simulink model "Copy_of_Channalizer_smoke_tmp"  (R2024a)
settings: Solver=VariableStepAuto  StartTime=0.0  StopTime=500  RelTol=1e-3
values from neighbouring files (symbols this model uses):
  X = simout    [outputPlots.m]
undefined symbols (not defined in the file or in its folder): Configured, DVB, es1, F, Initialized_retain_I, Pre, S, S2, vsva2488, xcvr1602
libraries: hdlBasic x21, hdlDSPIP x1, vmcUtilities x1
settings Model: Creator=nanumolu  LastModifiedBy=nanumolu

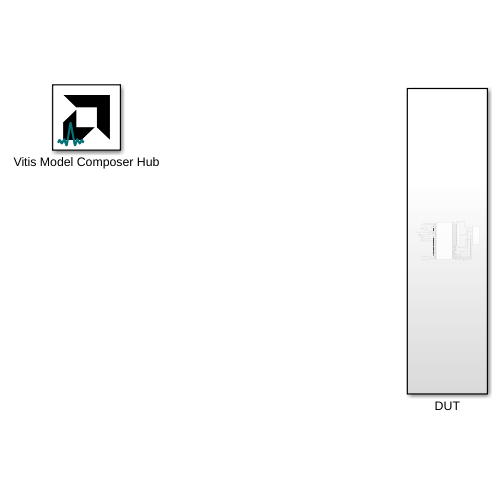
[thumbnail: Simulink's stored preview of the top-level diagram]
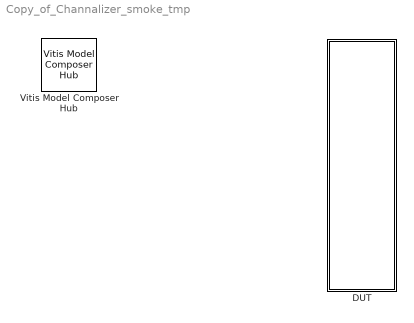
== system Copy_of_Channalizer_smoke_tmp ==
  DUT : Subsystem
  Vitis Model Composer Hub : vmcUtilities/Vitis Model Composer Hub  Tag=genX  CodeGeneration=off  SubsystemName=Channalizer_smoke_tmp  BlockHierPath=Channalizer_smoke_tmp  CompilationType=HDLCompilation  SubsystemType=HDLNode  ExportTypeV2=HDL Netlist  StartColumn=1  NumberOfColumns=1  TargetDirectory=./netlist_ldpc_vhd  exportDesign=on  analyzeDesign=off  validateDesignOnHw=off  ExportType=AI Engines  IpVendor=xilinx.com  IpLibrary=hls  IpVersion=1.0  IpHWLanguage=Verilog  AieCompilerOptions={}  AieSimulatorOptions={}  CreateTestbench=on  TestbenchStackSize=10  RunRtlSim=off  RunCSim=off  RunAieSim=off  AieSimTimeout=50000  RunAieSimProfiling=off  LaunchVitisAnalyzer=off  PlotOutput=off  RunX86Sim=off  X86SimTimeout=10  GenHwImage=off  GenLibadfXo=off  GenHwValidationCode=off  PlatformType=Not Specified  HwSystemType=Baremetal  HwValidationTarget=hw  ProjDevice=xcvr1602-vsva2488-2MP-e-S-es1  ProjDevicePart=xcvr1602-vsva2488-2MP-e-S-es1  AIEType=AIE  SamplePeriod=-1  ClockFrequency=200  DataPathParallelism=1  xilinxfamily=versalairfes1  part=xcvr1602  speed=-2MP-e-S-es1  package=vsva2488  directory=./netlist_ldpc_vhd  testbench=on  incr_netlist=off  synthesis_tool=Vivado  clock_wrapper=Clock Enables  dbl_ovrd=According to Block Masks  dcm_input_clock_period=10  sysclk_period=10  simulink_period=1  eval_field=0  IPInfoJsonString="{\"DUTSubsystemName\":\"Channalizer_smoke_tmp\",\"HDLSubsystem\":{\"SubsystemName\":\"Channalizer_smoke_tmp\",\"IPName\":\"Copy_of_hamilton_vrf_fft\",\"IPLibrary\":\"VMC\",\"IPVendor\":\"User Company\",\"IPVersion\":\"1.0\",\"TargetDirectory\":\"./netlist_ldpc_vhd\",\"SubsystemDir\":\"./netlist_ldpc_vhd/ip/Channalizer_smoke_tmp\",\"FreqHz\":\"100000000\"},\"SubsystemTag\":\"HDLNode\"}"  LogFileName=/proj/xhdhdstaff2/nanumolu/test/modelcomposer/hdl/regression/blocks/ip/RF_channelizer/smoke/Channalizer_smoke/netlist_ldpc_vhd/model_composer.log  NThreads=4  IPConfigFile=/tmp/vmctmp-3516168675900120850/Channalizer_smoke_tmp_ipconfig.json

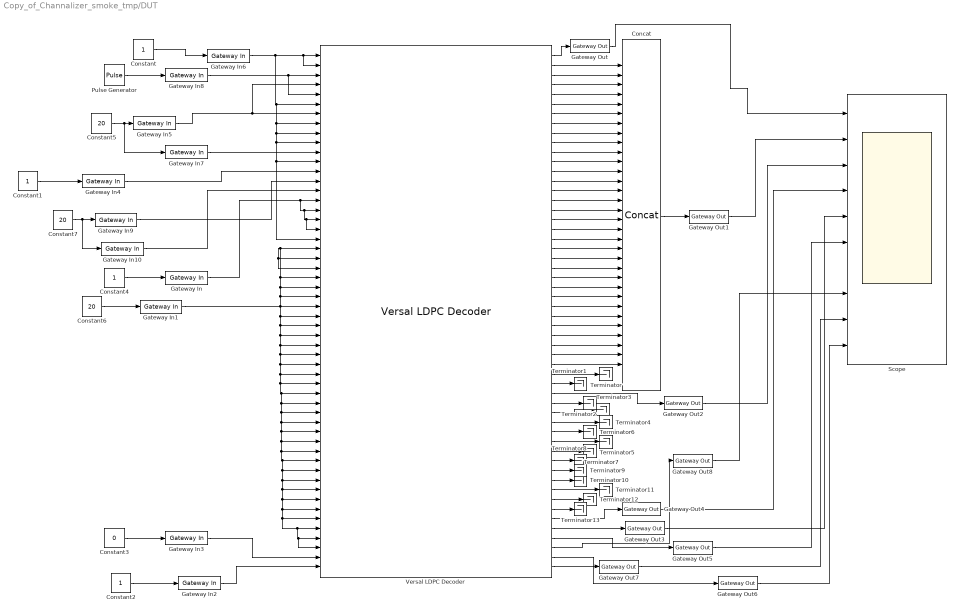
== system Copy_of_Channalizer_smoke_tmp/DUT ==
  Concat : hdlBasic/Concat  num_inputs=32  XmcBlockStatus=1  maskContainerNames=group1  block_type=concat  block_config=sysgen:Concat_config
  Constant : Constant  SampleTime=1/1e4
  Constant1 : Constant  SampleTime=1/1e4
  Constant2 : Constant  SampleTime=1
  Constant3 : Constant  Value=0  SampleTime=1
  Constant4 : Constant  SampleTime=1/1e4
  Constant5 : Constant  Value=20  SampleTime=1/1e4
  Constant6 : Constant  Value=20  SampleTime=1/1e4
  Constant7 : Constant  Value=20  SampleTime=1/1e4
  Gateway In : hdlBasic/Gateway In  gui_display_data_type=Fixed-point  arith_type=Unsigned  n_bits=1  bin_pt=0  preci_type=Single  exp_width=8  frac_width=24  rows=1  columns=1  quantization="Round  (unbiased: +/- Inf)"  overflow=Saturate  period=1  UseAsADC=off  ADCChannel='1'  interface=None  automatic_assignment=on  address_offset=hex2dec('00')  intf_name=''  intf_description=''  default_value=0  timing_constraint=None  locs_specified=off  LOCs={}  io_standard={}  inherit_from_input=off  hdl_port=on  XmcBlockStatus=1  maskContainerNames=group4  block_type=gatewayin  block_config=sysgen:gateway_in_config  block_width_w=590  block_height_w=620  block_width=640  block_height=850
  Gateway In1 : hdlBasic/Gateway In  gui_display_data_type=Fixed-point  arith_type=Signed (2's comp)  n_bits=8  bin_pt=2  preci_type=Single  exp_width=8  frac_width=24  rows=1  columns=1  quantization="Round  (unbiased: +/- Inf)"  overflow=Saturate  period=1  UseAsADC=off  ADCChannel='1'  interface=None  automatic_assignment=on  address_offset=hex2dec('00')  intf_name=''  intf_description=''  default_value=0  timing_constraint=None  locs_specified=off  LOCs={}  io_standard={}  inherit_from_input=off  hdl_port=on  XmcBlockStatus=1  maskContainerNames=group4  block_type=gatewayin  block_config=sysgen:gateway_in_config  block_width_w=590  block_height_w=620  block_width=640  block_height=850
  Gateway In10 : hdlBasic/Gateway In  gui_display_data_type=Fixed-point  arith_type=Unsigned  n_bits=6  bin_pt=0  preci_type=Single  exp_width=8  frac_width=24  rows=1  columns=1  quantization="Round  (unbiased: +/- Inf)"  overflow=Saturate  period=1  UseAsADC=off  ADCChannel='1'  interface=None  automatic_assignment=on  address_offset=hex2dec('00')  intf_name=''  intf_description=''  default_value=0  timing_constraint=None  locs_specified=off  LOCs={}  io_standard={}  inherit_from_input=off  hdl_port=on  XmcBlockStatus=1  maskContainerNames=group4  block_type=gatewayin  block_config=sysgen:gateway_in_config  block_width_w=590  block_height_w=620  block_width=640  block_height=850
  Gateway In2 : hdlBasic/Gateway In  gui_display_data_type=Boolean  arith_type=Boolean  n_bits=1  bin_pt=0  preci_type=Single  exp_width=8  frac_width=24  rows=1  columns=1  quantization="Round  (unbiased: +/- Inf)"  overflow=Saturate  period=1  UseAsADC=off  ADCChannel='1'  interface=None  automatic_assignment=on  address_offset=hex2dec('00')  intf_name=''  intf_description=''  default_value=0  timing_constraint=None  locs_specified=off  LOCs={}  io_standard={}  inherit_from_input=off  hdl_port=on  XmcBlockStatus=1  maskContainerNames=group4  block_type=gatewayin  block_config=sysgen:gateway_in_config  block_width_w=590  block_height_w=620  block_width=640  block_height=850
  Gateway In3 : hdlBasic/Gateway In  gui_display_data_type=Boolean  arith_type=Boolean  n_bits=1  bin_pt=0  preci_type=Single  exp_width=8  frac_width=24  rows=1  columns=1  quantization="Round  (unbiased: +/- Inf)"  overflow=Saturate  period=1  UseAsADC=off  ADCChannel='1'  interface=None  automatic_assignment=on  address_offset=hex2dec('00')  intf_name=''  intf_description=''  default_value=0  timing_constraint=None  locs_specified=off  LOCs={}  io_standard={}  inherit_from_input=off  hdl_port=on  XmcBlockStatus=1  maskContainerNames=group4  block_type=gatewayin  block_config=sysgen:gateway_in_config  block_width_w=590  block_height_w=620  block_width=640  block_height=850
  Gateway In4 : hdlBasic/Gateway In  gui_display_data_type=Fixed-point  arith_type=Unsigned  n_bits=8  bin_pt=0  preci_type=Single  exp_width=8  frac_width=24  rows=1  columns=1  quantization="Round  (unbiased: +/- Inf)"  overflow=Saturate  period=1  UseAsADC=off  ADCChannel='1'  interface=None  automatic_assignment=on  address_offset=hex2dec('00')  intf_name=''  intf_description=''  default_value=0  timing_constraint=None  locs_specified=off  LOCs={}  io_standard={}  inherit_from_input=off  hdl_port=on  XmcBlockStatus=1  maskContainerNames=group4  block_type=gatewayin  block_config=sysgen:gateway_in_config  block_width_w=590  block_height_w=620  block_width=640  block_height=850
  Gateway In5 : hdlBasic/Gateway In  gui_display_data_type=Fixed-point  arith_type=Signed (2's comp)  n_bits=18  bin_pt=0  preci_type=Single  exp_width=8  frac_width=24  rows=1  columns=1  quantization="Round  (unbiased: +/- Inf)"  overflow=Saturate  period=1  UseAsADC=off  ADCChannel='1'  interface=None  automatic_assignment=on  address_offset=hex2dec('00')  intf_name=''  intf_description=''  default_value=0  timing_constraint=None  locs_specified=off  LOCs={}  io_standard={}  inherit_from_input=off  hdl_port=on  XmcBlockStatus=1  maskContainerNames=group4  block_type=gatewayin  block_config=sysgen:gateway_in_config  block_width_w=590  block_height_w=620  block_width=640  block_height=850
  Gateway In6 : hdlBasic/Gateway In  gui_display_data_type=Boolean  arith_type=Boolean  n_bits=16  bin_pt=14  preci_type=Single  exp_width=8  frac_width=24  rows=1  columns=1  quantization="Round  (unbiased: +/- Inf)"  overflow=Saturate  period=1  UseAsADC=off  ADCChannel='1'  interface=None  automatic_assignment=on  address_offset=hex2dec('00')  intf_name=''  intf_description=''  default_value=0  timing_constraint=None  locs_specified=off  LOCs={}  io_standard={}  inherit_from_input=off  hdl_port=on  XmcBlockStatus=1  maskContainerNames=group4  block_type=gatewayin  block_config=sysgen:gateway_in_config  block_width_w=590  block_height_w=620  block_width=640  block_height=850
  Gateway In7 : hdlBasic/Gateway In  gui_display_data_type=Fixed-point  arith_type=Signed (2's comp)  n_bits=32  bin_pt=0  preci_type=Single  exp_width=8  frac_width=24  rows=1  columns=1  quantization="Round  (unbiased: +/- Inf)"  overflow=Saturate  period=1  UseAsADC=off  ADCChannel='1'  interface=None  automatic_assignment=on  address_offset=hex2dec('00')  intf_name=''  intf_description=''  default_value=0  timing_constraint=None  locs_specified=off  LOCs={}  io_standard={}  inherit_from_input=off  hdl_port=on  XmcBlockStatus=1  maskContainerNames=group4  block_type=gatewayin  block_config=sysgen:gateway_in_config  block_width_w=590  block_height_w=620  block_width=640  block_height=850
  Gateway In8 : hdlBasic/Gateway In  gui_display_data_type=Boolean  arith_type=Boolean  n_bits=16  bin_pt=14  preci_type=Single  exp_width=8  frac_width=24  rows=1  columns=1  quantization="Round  (unbiased: +/- Inf)"  overflow=Saturate  period=1  UseAsADC=off  ADCChannel='1'  interface=None  automatic_assignment=on  address_offset=hex2dec('00')  intf_name=''  intf_description=''  default_value=0  timing_constraint=None  locs_specified=off  LOCs={}  io_standard={}  inherit_from_input=off  hdl_port=on  XmcBlockStatus=1  maskContainerNames=group4  block_type=gatewayin  block_config=sysgen:gateway_in_config  block_width_w=590  block_height_w=620  block_width=640  block_height=850
  Gateway In9 : hdlBasic/Gateway In  gui_display_data_type=Fixed-point  arith_type=Unsigned  n_bits=7  bin_pt=0  preci_type=Single  exp_width=8  frac_width=24  rows=1  columns=1  quantization="Round  (unbiased: +/- Inf)"  overflow=Saturate  period=1  UseAsADC=off  ADCChannel='1'  interface=None  automatic_assignment=on  address_offset=hex2dec('00')  intf_name=''  intf_description=''  default_value=0  timing_constraint=None  locs_specified=off  LOCs={}  io_standard={}  inherit_from_input=off  hdl_port=on  XmcBlockStatus=1  maskContainerNames=group4  block_type=gatewayin  block_config=sysgen:gateway_in_config  block_width_w=590  block_height_w=620  block_width=640  block_height=850
  Gateway Out{,1..8} (9 alike) : hdlBasic/Gateway Out  inherit_from_input=off  bool_to_boolean=off  hdl_port=on  rows=1  columns=1  UseAsDAC=off  DACChannel='1'  interface=None  automatic_assignment=on  address_offset=hex2dec('00')  intf_name=''  intf_description=''  timing_constraint=None  locs_specified=off  LOCs={}  io_standard={}  XmcBlockStatus=1  maskContainerNames=group4  block_type=gatewayout  block_config=sysgen:gateway_out_config  block_width_w=590  block_height_w=620  block_width=620  block_height=750
  Pulse Generator : DiscretePulseGenerator  Period=500  PulseWidth=484  PhaseDelay=16
  Scope : Scope  NumInputPorts=10
  Terminator{,1..13} (14 alike) : Terminator
  Versal LDPC Decoder : hdlDSPIP/Versal LDPC Decoder  standard=DVB-S2(X)  ldpc_decode_algorithm_source=Initialized  ldpc_decode_algorithm_modifier_source=Initialized  ldpc_decode_sat_bits_source=Initialized  ldpc_decode_max_schedule_source=Initialized  ldpc_decode_code_definition='no_file_loaded'  ldpc_decode_overrides=on  ldpc_decode_algorithm=Normalized_MinSum  ldpc_decode_algorithm_modifier=12  ldpc_decode_sat_bits=6B  ldpc_decode_max_schedule=0  parameter_interface=Initialized_retain_I/F  enable_ifs=on  Interrupts=off  ecc_interrupts=None  bypass=off  din_interface=Pre-Configured  din_lanes=1  din_words_configuration=Fixed  din_words=32  dout_interface=Pre-Configured  dout_lanes=1  dout_words_configuration=Fixed  dout_words=32  throughput_utilization=100  ip_name=Versal LDPC Decoder  ip_version=1.0  dsptool_ready=false  ipcore_usecache=true  ipcore_useipmodelcache=true  wrapper_available=true  port_translation_map={ 'aclken' => 'en', aresetn' => 'rst' }  structural_sim=true  ipcore_do_not_force_period=true  XmcBlockStatus=1  maskContainerNames=tabcontainer1  block_type=versal_ldpc_v1_0  block_config=sysgen:rodinimport_config
  wires:
  Pulse Generator/1 -> Gateway In8/1
  Constant3/1 -> Gateway In3/1
  Constant/1 -> Gateway In6/1
  Constant1/1 -> Gateway In4/1
  Constant4/1 -> Gateway In/1
  Constant6/1 -> Gateway In1/1
  Gateway In8/1 -> Versal LDPC Decoder/5, Versal LDPC Decoder/3
  Gateway In6/1 -> Versal LDPC Decoder/6, Versal LDPC Decoder/8, Versal LDPC Decoder/9, Versal LDPC Decoder/10, Versal LDPC Decoder/20, Versal LDPC Decoder/12, Versal LDPC Decoder/2, Versal LDPC Decoder/1
  Gateway In5/1 -> Versal LDPC Decoder/7, Versal LDPC Decoder/4
  Gateway In4/1 -> Versal LDPC Decoder/13
  Gateway In9/1 -> Versal LDPC Decoder/14
  Gateway In10/1 -> Versal LDPC Decoder/15
  Gateway In/1 -> Versal LDPC Decoder/16, Versal LDPC Decoder/17, Versal LDPC Decoder/19, Versal LDPC Decoder/18
  Gateway In1/1 -> Versal LDPC Decoder/27, Versal LDPC Decoder/28, Versal LDPC Decoder/29, Versal LDPC Decoder/30, Versal LDPC Decoder/31, Versal LDPC Decoder/32, Versal LDPC Decoder/33, Versal LDPC Decoder/34, Versal LDPC Decoder/35, Versal LDPC Decoder/36, Versal LDPC Decoder/37, Versal LDPC Decoder/38, Versal LDPC Decoder/39, Versal LDPC Decoder/40, Versal LDPC Decoder/41, Versal LDPC Decoder/42, Versal LDPC Decoder/43, Versal LDPC Decoder/44, Versal LDPC Decoder/45, Versal LDPC Decoder/46, Versal LDPC Decoder/47, Versal LDPC Decoder/48, Versal LDPC Decoder/49, Versal LDPC Decoder/50, Versal LDPC Decoder/52, Versal LDPC Decoder/51, Versal LDPC Decoder/26, Versal LDPC Decoder/25, Versal LDPC Decoder/24, Versal LDPC Decoder/21, Versal LDPC Decoder/23, Versal LDPC Decoder/22
  Gateway In3/1 -> Versal LDPC Decoder/53
  Gateway In2/1 -> Versal LDPC Decoder/54
  Constant2/1 -> Gateway In2/1
  Gateway In7/1 -> Versal LDPC Decoder/11
  Versal LDPC Decoder/1 -> Gateway Out/1
  Versal LDPC Decoder/2 -> Concat/1
  Versal LDPC Decoder/3 -> Concat/2
  Versal LDPC Decoder/4 -> Concat/3
  Versal LDPC Decoder/5 -> Concat/4
  Versal LDPC Decoder/6 -> Concat/5
  Versal LDPC Decoder/7 -> Concat/6
  Versal LDPC Decoder/8 -> Concat/7
  Versal LDPC Decoder/9 -> Concat/8
  Versal LDPC Decoder/10 -> Concat/9
  Versal LDPC Decoder/11 -> Concat/10
  Versal LDPC Decoder/12 -> Concat/11
  Versal LDPC Decoder/13 -> Concat/12
  Versal LDPC Decoder/14 -> Concat/13
  Versal LDPC Decoder/15 -> Concat/14
  Versal LDPC Decoder/16 -> Concat/15
  Versal LDPC Decoder/17 -> Concat/16
  Versal LDPC Decoder/18 -> Concat/17
  Versal LDPC Decoder/19 -> Concat/18
  Versal LDPC Decoder/20 -> Concat/19
  Versal LDPC Decoder/21 -> Concat/20
  Versal LDPC Decoder/22 -> Concat/21
  Versal LDPC Decoder/23 -> Concat/22
  Versal LDPC Decoder/24 -> Concat/23
  Versal LDPC Decoder/25 -> Concat/24
  Versal LDPC Decoder/26 -> Concat/25
  Versal LDPC Decoder/27 -> Concat/26
  Versal LDPC Decoder/28 -> Concat/27
  Versal LDPC Decoder/29 -> Concat/28
  Versal LDPC Decoder/30 -> Concat/29
  Versal LDPC Decoder/31 -> Concat/30
  Versal LDPC Decoder/32 -> Concat/31
  Versal LDPC Decoder/33 -> Concat/32
  Concat/1 -> Gateway Out1/1
  Versal LDPC Decoder/34 -> Terminator/1
  Versal LDPC Decoder/36 -> Gateway Out2/1
  Versal LDPC Decoder/35 -> Terminator1/1
  Versal LDPC Decoder/37 -> Terminator2/1
  Versal LDPC Decoder/50 -> Gateway Out3/1
  Versal LDPC Decoder/49 -> Gateway Out4/1
  Versal LDPC Decoder/51 -> Gateway Out5/1
  Versal LDPC Decoder/53 -> Gateway Out6/1
  Versal LDPC Decoder/54 -> Gateway Out7/1
  Versal LDPC Decoder/52 -> Gateway Out8/1
  Versal LDPC Decoder/38 -> Terminator3/1
  Versal LDPC Decoder/39 -> Terminator4/1
  Versal LDPC Decoder/41 -> Terminator5/1
  Versal LDPC Decoder/40 -> Terminator6/1
  Versal LDPC Decoder/42 -> Terminator7/1
  Versal LDPC Decoder/43 -> Terminator8/1
  Versal LDPC Decoder/44 -> Terminator9/1
  Versal LDPC Decoder/45 -> Terminator10/1
  Versal LDPC Decoder/46 -> Terminator11/1
  Versal LDPC Decoder/47 -> Terminator12/1
  Versal LDPC Decoder/48 -> Terminator13/1
  Gateway Out/1 -> Scope/1
  Gateway Out1/1 -> Scope/2
  Gateway Out2/1 -> Scope/3
  Gateway Out4/1 -> Scope/4
  Gateway Out3/1 -> Scope/5
  Gateway Out5/1 -> Scope/6
  Gateway Out6/1 -> Scope/10
  Gateway Out7/1 -> Scope/9
  Gateway Out8/1 -> Scope/8
  Constant5/1 -> Gateway In7/1, Gateway In5/1
  Constant7/1 -> Gateway In10/1, Gateway In9/1
